simulink model "HX_independentSISO_2023b_mdl"  (R2023b)
settings: Solver=ode4  StartTime=0  StopTime=300  FixedStep=0.001  RelTol=1e-3
settings Model: Creator=mohammadodeh  LastModifiedBy=mohammadodeh

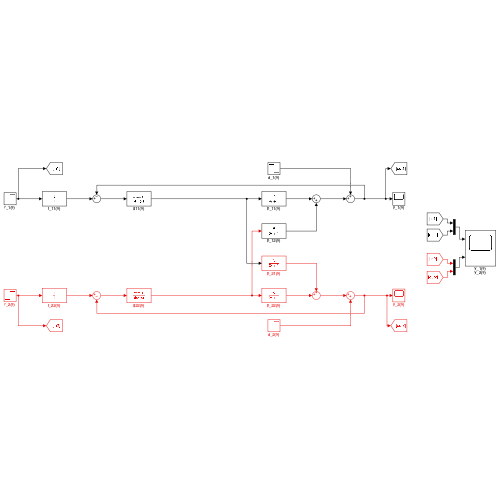
[thumbnail: Simulink's stored preview of the top-level diagram]
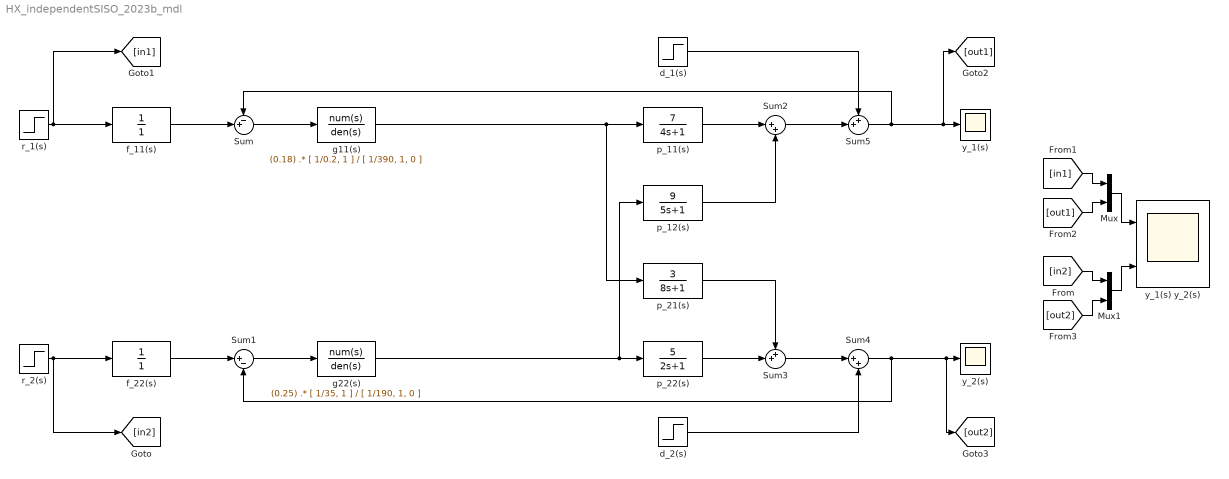
== system HX_independentSISO_2023b_mdl ==
  Mux : Mux  Inputs=2
  Mux1 : Mux  Inputs=2
  Sum : Sum  Inputs=-+|
  Sum1 : Sum  Inputs=|+-
  Sum2 : Sum  Inputs=|++
  Sum3 : Sum  Inputs=++|
  Sum4 : Sum  Inputs=|++
  Sum5 : Sum  Inputs=++|
  d_1(s) : Step  Time=250  After=-1  SampleTime=0
  d_2(s) : Step  Time=120  After=0.25  SampleTime=0
  f_11(s) : TransferFcn  Numerator=1  Denominator=1
  f_22(s) : TransferFcn  Numerator=1  Denominator=1
  g11(s) : TransferFcn  Numerator=(0.18) .* [ 1/0.2, 1 ]  Denominator=[ 1/390, 1, 0 ]
  g22(s) : TransferFcn  Numerator=(0.25) .* [ 1/35, 1 ]  Denominator=[ 1/190, 1, 0 ]
  p_11(s) : TransferFcn  Numerator=7  Denominator=[4, 1]
  p_12(s) : TransferFcn  Numerator=9  Denominator=[5, 1]
  p_21(s) : TransferFcn  Numerator=3  Denominator=[8, 1]
  p_22(s) : TransferFcn  Numerator=5  Denominator=[2, 1]
  r_1(s) : Step  Time=20  SampleTime=0
  r_2(s) : Step  Time=170  SampleTime=0
  y_1(s) : Scope
  y_1(s) y_2(s) : Scope  NumInputPorts=2
  y_2(s) : Scope
  wires:
  f_11(s)/1 -> Sum/2
  Sum/1 -> g11(s)/1
  f_22(s)/1 -> Sum1/1
  Sum1/1 -> g22(s)/1
  r_1(s)/1 -> [in1], f_11(s)/1
  r_2(s)/1 -> f_22(s)/1, [in2]
  Sum4/1 -> [out2], y_2(s)/1, Sum1/2
  d_1(s)/1 -> Sum5/1
  Sum5/1 -> [out1], y_1(s)/1, Sum/1
  p_21(s)/1 -> Sum3/1
  p_12(s)/1 -> Sum2/2
  d_2(s)/1 -> Sum4/2
  p_22(s)/1 -> Sum3/2
  Sum3/1 -> Sum4/1
  p_11(s)/1 -> Sum2/1
  Sum2/1 -> Sum5/2
  g11(s)/1 -> p_21(s)/1, p_11(s)/1
  g22(s)/1 -> p_12(s)/1, p_22(s)/1
  Mux/1 -> y_1(s) y_2(s)/1
  Mux1/1 -> y_1(s) y_2(s)/2
  [in2] -> Mux1/1
  [in1] -> Mux/1
  [out1] -> Mux/2
  [out2] -> Mux1/2
